simulink model "task4_1"  (R2024b)
settings: Solver=VariableStepAuto  StartTime=0.0  StopTime=10  RelTol=1e-3
values from neighbouring files (symbols this model uses):
  J = 9.0e-7    (= 9e-07)    [ball_beam_properties.m]
  m = 0.01    [ball_beam_properties.m]
  R = 0.015    [ball_beam_properties.m]
undefined symbols (not defined in the file or in its folder): g
settings Model: Creator=ASUS  LastModifiedBy=ASUS

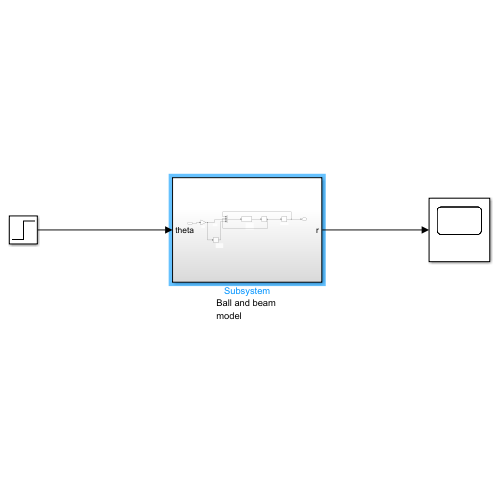
[thumbnail: Simulink's stored preview of the top-level diagram]
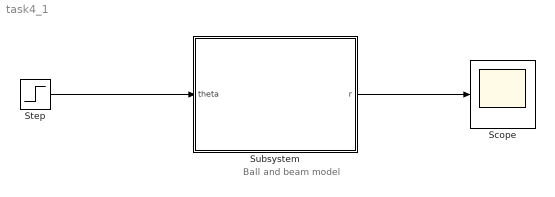
== system task4_1 ==
  note: Ball and beam
      | model
  Scope : Scope
  Step : Step  Time=0  SampleTime=0
  Subsystem : Subsystem
  wires:
  Step/1 -> Subsystem/1(theta)
  Subsystem/1(r) -> Scope/1

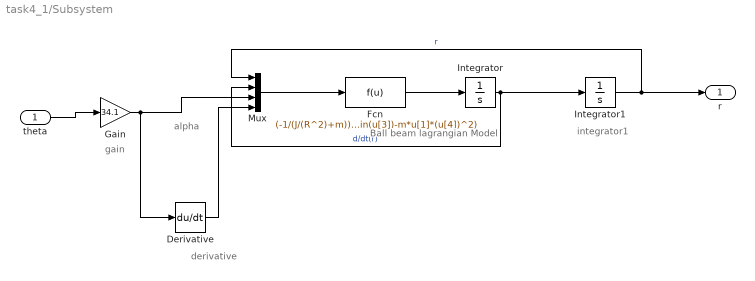
== system task4_1/Subsystem ==
  note: derivative
  note: alpha
  note: integrator1
  note: Ball beam
      | lagrangian
      | Model
  note: gain
  theta : Inport
  Derivative : Derivative
  Fcn : Fcn  Expr=(-1/(J/(R^2)+m))*(m*g*sin(u[3])-m*u[1]*(u[4])^2)
  Gain : Gain  Gain=34.1
  Integrator : Integrator
  Integrator1 : Integrator
  Mux : Mux
  r : Outport
  wires:
  Gain/1 -> Derivative/1, Mux/3
  Derivative/1 -> Mux/4
  Integrator1/1 -> Mux/1, r/1  "r"
  theta/1 -> Gain/1
  Fcn/1 -> Integrator/1
  Mux/1 -> Fcn/1
  Integrator/1 -> Mux/2, Integrator1/1  "d/dt(r)"
